simulink model "Control_Block_2"  (R2021b)
settings: Solver=FixedStepAuto  StartTime=0.0  StopTime=end_time  FixedStep=dt  RelTol=1e-3
values from neighbouring files (symbols this model uses):
  Area = pi() * r0^2    [Main_PD_Control.m]
  Cd = 0.42    [Main_PD_Control.m]
  dt = 0.01    [Main_PD_Control.m]
  K_d = 10    [Main_PD_Control.m]
  K_p = 100    [Main_PD_Control.m]
  rho = 1000    [Main_PD_Control.m]
settings Model: Creator=zhong  LastModifiedBy=zhong

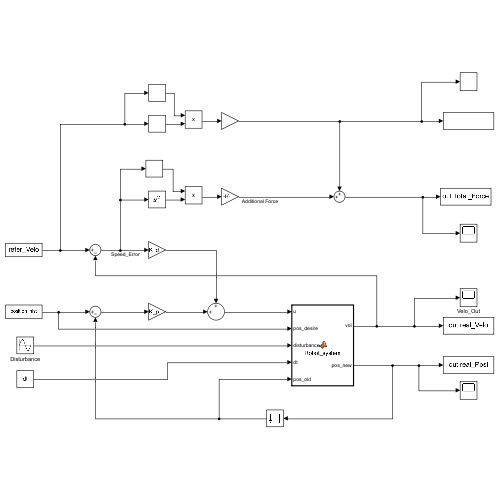
[thumbnail: Simulink's stored preview of the top-level diagram]
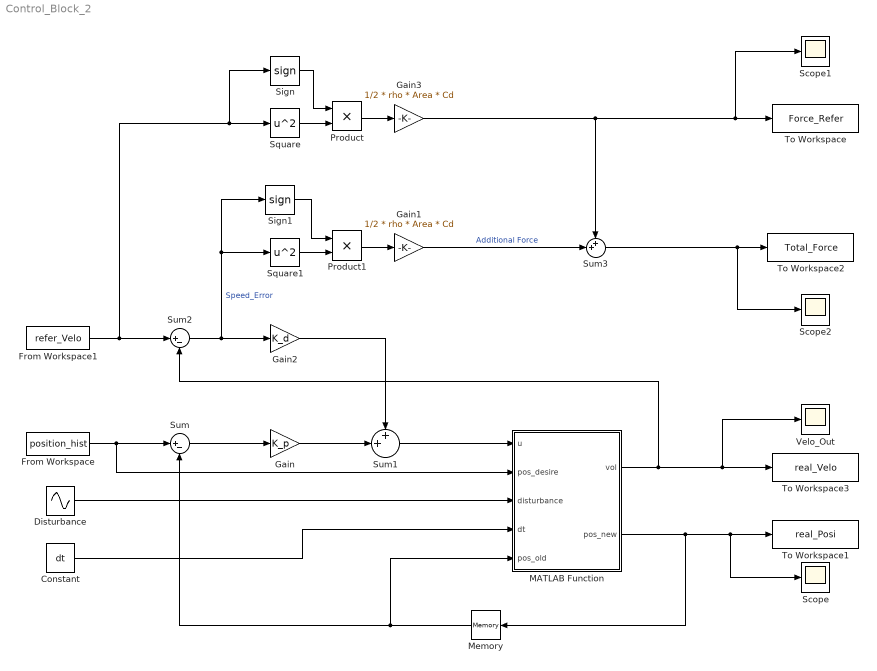
== system Control_Block_2 ==
  Constant : Constant  Value=dt
  Disturbance : Sin  Amplitude=2  Frequency=10  SampleTime=0
  From Workspace : FromWorkspace  VariableName=position_hist
  From Workspace1 : FromWorkspace  VariableName=refer_Velo
  Gain : Gain  Gain=K_p
  Gain1 : Gain  Gain=1/2 * rho * Area * Cd
  Gain2 : Gain  Gain=K_d
  Gain3 : Gain  Gain=1/2 * rho * Area * Cd
  MATLAB Function : MATLAB Function  TreatAsAtomicUnit=on
  Memory : Memory
  Product : Product
  Product1 : Product
  Scope : Scope
  Scope1 : Scope
  Scope2 : Scope
  Sign : Signum
  Sign1 : Signum
  Square : Math  Operator=square  SaturateOnIntegerOverflow=on
  Square1 : Math  Operator=square  SaturateOnIntegerOverflow=on
  Sum : Sum  Inputs=|+-
  Sum1 : Sum  Inputs=++|
  Sum2 : Sum  Inputs=|+-
  Sum3 : Sum  Inputs=++|
  To Workspace : ToWorkspace  VariableName=Force_Refer  SaveFormat=Timeseries  SampleTime=-1
  To Workspace1 : ToWorkspace  VariableName=real_Posi  SaveFormat=Timeseries  SampleTime=-1
  To Workspace2 : ToWorkspace  VariableName=Total_Force  SaveFormat=Timeseries  SampleTime=-1
  To Workspace3 : ToWorkspace  VariableName=real_Velo  SaveFormat=Timeseries  SampleTime=-1
  Velo_Out : Scope
  wires:
  From Workspace/1 -> MATLAB Function/2(pos_desire), Sum/1
  Sum/1 -> Gain/1
  Gain/1 -> Sum1/2
  Sum2/1 -> Sign1/1, Square1/1, Gain2/1  "Speed_Error"
  Gain2/1 -> Sum1/1
  Sum1/1 -> MATLAB Function/1(u)
  From Workspace1/1 -> Sum2/1, Sign/1, Square/1
  Sum3/1 -> Scope2/1, To Workspace2/1
  Constant/1 -> MATLAB Function/4(dt)
  Disturbance/1 -> MATLAB Function/3(disturbance)
  MATLAB Function/2(pos_new) -> Memory/1, Scope/1, To Workspace1/1
  Memory/1 -> MATLAB Function/5(pos_old), Sum/2
  MATLAB Function/1(vol) -> Sum2/2, Velo_Out/1, To Workspace3/1
  Gain3/1 -> Sum3/1, Scope1/1, To Workspace/1
  Gain1/1 -> Sum3/2  "Additional Force"
  Square/1 -> Product/2
  Sign/1 -> Product/1
  Product/1 -> Gain3/1
  Sign1/1 -> Product1/1
  Square1/1 -> Product1/2
  Product1/1 -> Gain1/1

== matlab function Control_Block_2/MATLAB Function ==
  data: vol output; u input; pos_desire input; disturbance input; dt input; pos_old input; pos_new output
function [vol,pos_new] = Robot_system(u,pos_desire,disturbance,dt,pos_old)

pos_new = pos_desire + u + disturbance;

vol = (pos_new - pos_old)/dt;
